simulink model "model1"  (R2024b)
settings: Solver=VariableStepAuto  StartTime=0.0  StopTime=10.0  RelTol=1e-3
settings Model: Creator=Mehmet  LastModifiedBy=Mehmet

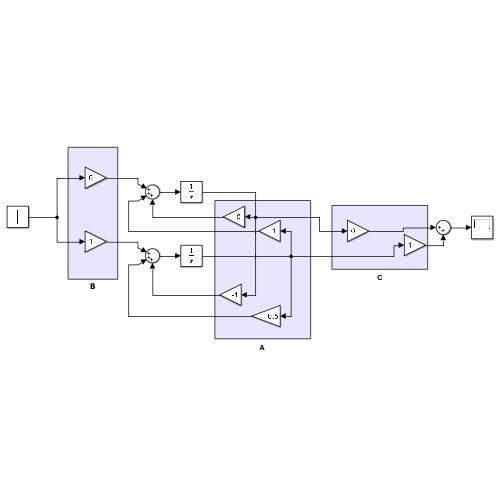
[thumbnail: Simulink's stored preview of the top-level diagram]
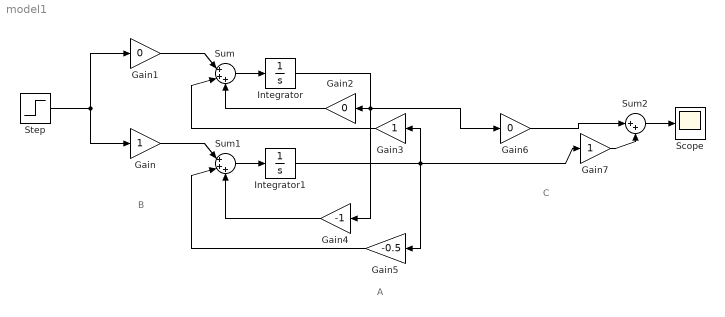
== system model1 ==
  note: C
  note: B
  note: A
  Gain : Gain
  Gain1 : Gain  Gain=0
  Gain2 : Gain  Gain=0
  Gain3 : Gain
  Gain4 : Gain  Gain=-1
  Gain5 : Gain  Gain=-0.5
  Gain6 : Gain  Gain=0
  Gain7 : Gain
  Integrator : Integrator
  Integrator1 : Integrator
  Scope : Scope
  Step : Step  SampleTime=0
  Sum : Sum  Inputs=|+++
  Sum1 : Sum  Inputs=|+++
  Sum2 : Sum  Inputs=|++
  wires:
  Gain1/1 -> Sum/1
  Gain/1 -> Sum1/1
  Gain2/1 -> Sum/3
  Gain3/1 -> Sum/2
  Gain4/1 -> Sum1/3
  Gain5/1 -> Sum1/2
  Sum1/1 -> Integrator1/1
  Integrator/1 -> Gain6/1, Gain4/1, Gain2/1
  Integrator1/1 -> Gain3/1, Gain7/1, Gain5/1
  Gain6/1 -> Sum2/1
  Gain7/1 -> Sum2/2
  Step/1 -> Gain1/1, Gain/1
  Sum2/1 -> Scope/1
  Sum/1 -> Integrator/1
